simulink model "Primerpunto"  (R2016b)
settings: Solver=VariableStepAuto  StartTime=0.0  StopTime=10  RelTol=1e-3  EnableMultiTasking=on
libraries: commutil2 x4, commsrccod2 x2, dspquant2 x2, dspobslib x1, dspvision x1
settings Model: Creator=pc  LastModifiedBy=JULIAN CAMILO
settings DataIOCC: LimitDataPoints=on
settings OptimizationCC: LifeSpan=inf
settings DebuggingCC: AllowSymbolicDim=off  SFUnexpectedBacktrackingDiag=warning  SFNoUnconditionalDefaultTransitionDiag=warning  SFExecutionAtInitializationDiag=none
settings ModelReferenceCC: PropagateSignalLabelsOutOfModel=off
settings GRTTargetCC: TargetLangStandard=C89/C90 (ANSI)
settings ConfigComp: CovMetricSettings=dw  CovHtmlReporting=on  CovSaveCumulativeToWorkspaceVar=on  CovSaveSingleToWorkspaceVar=on  CovExternalEMLEnable=off

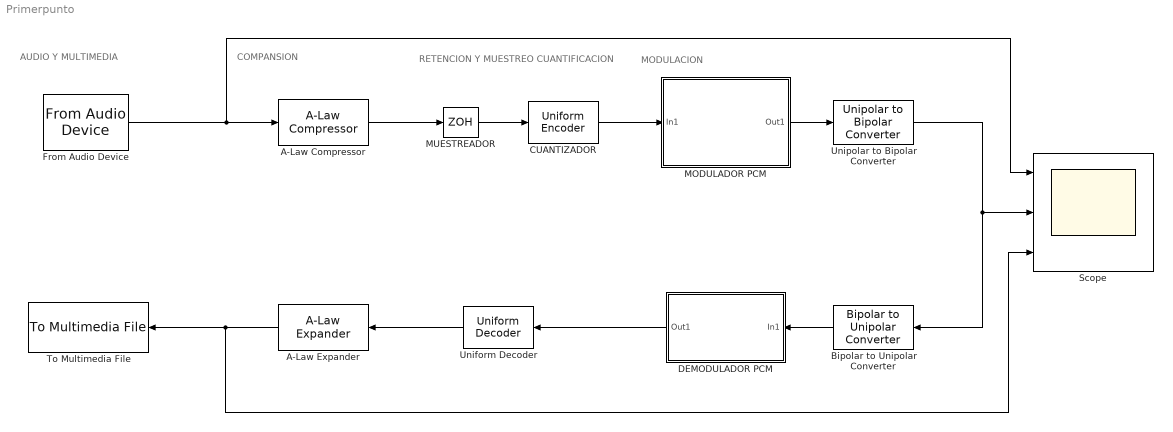
== system Primerpunto ==
  note: RETENCION Y MUESTREO
      | CUANTIFICACION
  note: COMPANSION
  note: AUDIO Y
      | MULTIMEDIA
  note: MODULACION
  A-Law Compressor : commsrccod2/A-Law Compressor  A=87.6  V=1
  A-Law Expander : commsrccod2/A-Law Expander  A=87.6  V=1
  Bipolar to Unipolar Converter : commutil2/Bipolar to Unipolar Converter  M=2  polarity=Positive  dataType=int8
  CUANTIZADOR : dspquant2/Uniform Encoder  peak=1  bits=8  otype=Unsigned integer
  DEMODULADOR PCM : Subsystem
  From Audio Device : dspobslib/From Audio Device  deviceName=Default  numChannels=1  sampleRate=44100  deviceDatatype=Determine from output data type  autoBufferSize=on  bufferSize=4096  queueDuration=0.1  frameSize=1  outputDatatype=double  defaultInputChannelMapping=on  inputChannelMapping=1:2  outputNumOverrunSamples=off  OutputFrames=off
  MODULADOR PCM : Subsystem
  MUESTREADOR : ZeroOrderHold  SampleTime=1/(8*4000)
  Scope : Scope  NumInputPorts=3
  To Multimedia File : dspvision/To Multimedia File  outputFilename=output.wav  streamSelection=Audio only  videoCompressor=None (uncompressed)  audioCompressor=None (uncompressed)  imagePorts=Separate color signals  fileType=WAV  audioDatatype=16-bit integer  fourcc=RGB  videoQuality=75  mj2000CompFactor=10
  Uniform Decoder : dspquant2/Uniform Decoder  peak=1  bits=8  overflowMode=Saturate  otype=Double
  Unipolar to Bipolar Converter : commutil2/Unipolar to Bipolar Converter  M=2  polarity=Positive  dataType=Inherit via internal rule
  wires:
  MUESTREADOR/1 -> CUANTIZADOR/1
  From Audio Device/1 -> A-Law Compressor/1, Scope/1
  A-Law Expander/1 -> Scope/3, To Multimedia File/1
  A-Law Compressor/1 -> MUESTREADOR/1
  Uniform Decoder/1 -> A-Law Expander/1
  Unipolar to Bipolar Converter/1 -> Scope/2, Bipolar to Unipolar Converter/1
  MODULADOR PCM/1(Out1) -> Unipolar to Bipolar Converter/1
  Bipolar to Unipolar Converter/1 -> DEMODULADOR PCM/1(In1)
  CUANTIZADOR/1 -> MODULADOR PCM/1(In1)
  DEMODULADOR PCM/1(Out1) -> Uniform Decoder/1

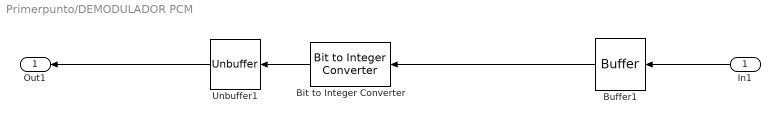
== system Primerpunto/DEMODULADOR PCM ==
  In1 : Inport
  Bit to Integer Converter : commutil2/Bit to Integer Converter  nbits=8  bitOrder=MSB first  signedOutputValues=Unsigned  outDtype=uint8  outDtypeSigned=Inherit via internal rule
  Buffer1 : Buffer  N=3*8  TreatMby1Signals=One channel  OutputFrames=off
  Unbuffer1 : Unbuffer  SampleBasedProcessing=Same as frame based
  Out1 : Outport
  wires:
  Buffer1/1 -> Bit to Integer Converter/1
  In1/1 -> Buffer1/1
  Bit to Integer Converter/1 -> Unbuffer1/1
  Unbuffer1/1 -> Out1/1

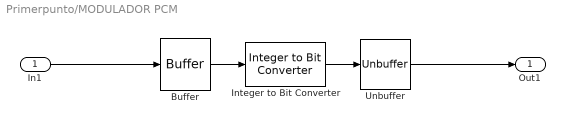
== system Primerpunto/MODULADOR PCM ==
  In1 : Inport
  Buffer : Buffer  N=3  TreatMby1Signals=One channel  OutputFrames=off
  Integer to Bit Converter : commutil2/Integer to Bit Converter  nbits=8  signedInputValues=Unsigned  bitOrder=MSB first  outDtype=Inherit via internal rule
  Unbuffer : Unbuffer  SampleBasedProcessing=Same as frame based
  Out1 : Outport
  wires:
  Integer to Bit Converter/1 -> Unbuffer/1
  Unbuffer/1 -> Out1/1
  Buffer/1 -> Integer to Bit Converter/1
  In1/1 -> Buffer/1
